simulink model "NLSys"  (R2018b)
settings: Solver=VariableStepAuto  StartTime=0.0  StopTime=10.0  RelTol=1e-3
settings Model: Creator=Jyot Buch  LastModifiedBy=Jyot Buch

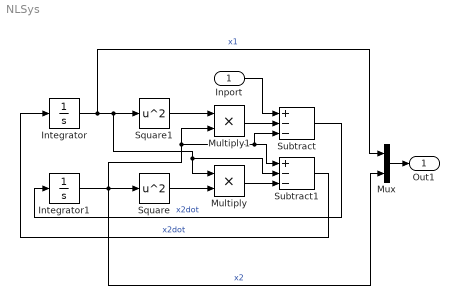
== system NLSys ==
  Inport : Inport
  Integrator : Integrator
  Integrator1 : Integrator
  Multiply : Product
  Multiply1 : Product
  Mux : Mux  Inputs=2
  Square : Math  Operator=square  SaturateOnIntegerOverflow=on
  Square1 : Math  Operator=square  SaturateOnIntegerOverflow=on
  Subtract : Sum  Inputs=+--
  Subtract1 : Sum  Inputs=+--
  Out1 : Outport
  wires:
  Integrator/1 -> Mux/1, Subtract1/2, Multiply/1, Square1/1  "x1"
  Integrator1/1 -> Multiply1/2, Subtract1/1, Subtract/3, Mux/2, Square/1  "x2"
  Square1/1 -> Multiply1/1
  Square/1 -> Multiply/2
  Multiply/1 -> Subtract1/3
  Multiply1/1 -> Subtract/2
  Inport/1 -> Subtract/1
  Subtract/1 -> Integrator1/1  "x2dot"
  Subtract1/1 -> Integrator/1  "x2dot"
  Mux/1 -> Out1/1
